simulink model "TST_HLSDem_SelectParameter"  (R2016b)
settings: Solver=FixedStepDiscrete  StartTime=0.0  StopTime=simTime  FixedStep=sampleTime  RelTol=1e-3
values from neighbouring files (symbols this model uses):
  testCase = 1    [initTST_HLSDem_SelectParameter_001.m]    (also in initTST_HLSDem_SelectParameter_002.m = 2; initTST_HLSDem_SelectParameter_003.m = 3; initTST_HLSDem_SelectParameter_004.m = 4; initTST_HLSDem_SelectParameter_005.m = 5)
libraries: simulink x146, UnitTest_Lib x140
(part 3 of 4)

== system TST_HLSDem_SelectParameter/simulationInput/testSignals_R002 ==
  BC : BusCreator  Inputs=37
  spec_CEngDsT_t : FromWorkspace  VariableName=testSig_CEngDsT_t  Interpolate=off  OutputAfterFinalValue=Holding final value
  spec_EngDa_tEng : FromWorkspace  VariableName=testSig_EngDa_tEng  Interpolate=off  OutputAfterFinalValue=Holding final value
  spec_Epm_nEng : FromWorkspace  VariableName=testSig_Epm_nEng  Interpolate=off  OutputAfterFinalValue=Holding final value
  spec_GlbDa_rTrqTot : FromWorkspace  VariableName=testSig_GlbDa_rTrqTot  Interpolate=off  OutputAfterFinalValue=Holding final value
  spec_HLSDem_IWinNegHiCurr_mp : FromWorkspace  VariableName=testSig_HLSDem_IWinNegHiCurr_mp  Interpolate=off  OutputAfterFinalValue=Holding final value
  spec_HLSDem_IWinNegLoCurr_mp : FromWorkspace  VariableName=testSig_HLSDem_IWinNegLoCurr_mp  Interpolate=off  OutputAfterFinalValue=Holding final value
  spec_HLSDem_IWinPosHiCurr_mp : FromWorkspace  VariableName=testSig_HLSDem_IWinPosHiCurr_mp  Interpolate=off  OutputAfterFinalValue=Holding final value
  spec_HLSDem_IWinPosLoCurr_mp : FromWorkspace  VariableName=testSig_HLSDem_IWinPosLoCurr_mp  Interpolate=off  OutputAfterFinalValue=Holding final value
  spec_HLSDem_InrtVehCurr : FromWorkspace  VariableName=testSig_HLSDem_InrtVehCurr  Interpolate=off  OutputAfterFinalValue=Holding final value
  spec_HLSDem_KiHiCurr_mp : FromWorkspace  VariableName=testSig_HLSDem_KiHiCurr_mp  Interpolate=off  OutputAfterFinalValue=Holding final value
  spec_HLSDem_KiLoCurr_mp : FromWorkspace  VariableName=testSig_HLSDem_KiLoCurr_mp  Interpolate=off  OutputAfterFinalValue=Holding final value
  spec_HLSDem_KiNegHiCurr_mp : FromWorkspace  VariableName=testSig_HLSDem_KiNegHiCurr_mp  Interpolate=off  OutputAfterFinalValue=Holding final value
  spec_HLSDem_KiNegLoCurr_mp : FromWorkspace  VariableName=testSig_HLSDem_KiNegLoCurr_mp  Interpolate=off  OutputAfterFinalValue=Holding final value
  spec_HLSDem_KiPosHiCurr_mp : FromWorkspace  VariableName=testSig_HLSDem_KiPosHiCurr_mp  Interpolate=off  OutputAfterFinalValue=Holding final value
  spec_HLSDem_KiPosLoCurr_mp : FromWorkspace  VariableName=testSig_HLSDem_KiPosLoCurr_mp  Interpolate=off  OutputAfterFinalValue=Holding final value
  spec_HLSDem_KpHiCurr_mp : FromWorkspace  VariableName=testSig_HLSDem_KpHiCurr_mp  Interpolate=off  OutputAfterFinalValue=Holding final value
  spec_HLSDem_KpLoCurr_mp : FromWorkspace  VariableName=testSig_HLSDem_KpLoCurr_mp  Interpolate=off  OutputAfterFinalValue=Holding final value
  spec_HLSDem_KpNegHiCurr_mp : FromWorkspace  VariableName=testSig_HLSDem_KpNegHiCurr_mp  Interpolate=off  OutputAfterFinalValue=Holding final value
  spec_HLSDem_KpNegLoCurr_mp : FromWorkspace  VariableName=testSig_HLSDem_KpNegLoCurr_mp  Interpolate=off  OutputAfterFinalValue=Holding final value
  spec_HLSDem_KpPosHiCurr_mp : FromWorkspace  VariableName=testSig_HLSDem_KpPosHiCurr_mp  Interpolate=off  OutputAfterFinalValue=Holding final value
  spec_HLSDem_KpPosLoCurr_mp : FromWorkspace  VariableName=testSig_HLSDem_KpPosLoCurr_mp  Interpolate=off  OutputAfterFinalValue=Holding final value
  spec_HLSDem_PWinNegHiCurr_mp : FromWorkspace  VariableName=testSig_HLSDem_PWinNegHiCurr_mp  Interpolate=off  OutputAfterFinalValue=Holding final value
  spec_HLSDem_PWinNegLoCurr_mp : FromWorkspace  VariableName=testSig_HLSDem_PWinNegLoCurr_mp  Interpolate=off  OutputAfterFinalValue=Holding final value
  spec_HLSDem_PWinPosHiCurr_mp : FromWorkspace  VariableName=testSig_HLSDem_PWinPosHiCurr_mp  Interpolate=off  OutputAfterFinalValue=Holding final value
  spec_HLSDem_PWinPosLoCurr_mp : FromWorkspace  VariableName=testSig_HLSDem_PWinPosLoCurr_mp  Interpolate=off  OutputAfterFinalValue=Holding final value
  spec_HLSDem_dnAccLim : FromWorkspace  VariableName=testSig_HLSDem_dnAccLim  Interpolate=off  OutputAfterFinalValue=Holding final value
  spec_HLSDem_dnDeclLim : FromWorkspace  VariableName=testSig_HLSDem_dnDeclLim  Interpolate=off  OutputAfterFinalValue=Holding final value
  spec_HLSDem_facFdbkHi : FromWorkspace  VariableName=testSig_HLSDem_facFdbkHi  Interpolate=off  OutputAfterFinalValue=Holding final value
  spec_HLSDem_facFdbkLo : FromWorkspace  VariableName=testSig_HLSDem_facFdbkLo  Interpolate=off  OutputAfterFinalValue=Holding final value
  spec_HLSDem_facFdbkTrqLosHi : FromWorkspace  VariableName=testSig_HLSDem_facFdbkTrqLosHi  Interpolate=off  OutputAfterFinalValue=Holding final value
  spec_HLSDem_facFdbkTrqLosLo : FromWorkspace  VariableName=testSig_HLSDem_facFdbkTrqLosLo  Interpolate=off  OutputAfterFinalValue=Holding final value
  spec_HLSDem_tiFltTrqLosEstCurr : FromWorkspace  VariableName=testSig_HLSDem_tiFltTrqLosEstCurr  Interpolate=off  OutputAfterFinalValue=Holding final value
  spec_Oil_tSwmp : FromWorkspace  VariableName=testSig_Oil_tSwmp  Interpolate=off  OutputAfterFinalValue=Holding final value
  spec_PT_rGrip : FromWorkspace  VariableName=testSig_PT_rGrip  Interpolate=off  OutputAfterFinalValue=Holding final value
  spec_PthLead_trqInrCurr : FromWorkspace  VariableName=testSig_PthLead_trqInrCurr  Interpolate=off  OutputAfterFinalValue=Holding final value
  spec_PthLead_trqInrLead : FromWorkspace  VariableName=testSig_PthLead_trqInrLead  Interpolate=off  OutputAfterFinalValue=Holding final value
  spec_PthSet_trqInrSet : FromWorkspace  VariableName=testSig_PthSet_trqInrSet  Interpolate=off  OutputAfterFinalValue=Holding final value
  testSignals : Outport
  wires:
  BC/1 -> testSignals/1
  spec_Epm_nEng/1 -> BC/1  "testSig_Epm_nEng"
  spec_PT_rGrip/1 -> BC/2  "testSig_PT_rGrip"
  spec_GlbDa_rTrqTot/1 -> BC/3  "testSig_GlbDa_rTrqTot"
  spec_PthSet_trqInrSet/1 -> BC/4  "testSig_PthSet_trqInrSet"
  spec_PthLead_trqInrCurr/1 -> BC/5  "testSig_PthLead_trqInrCurr"
  spec_PthLead_trqInrLead/1 -> BC/6  "testSig_PthLead_trqInrLead"
  spec_CEngDsT_t/1 -> BC/7  "testSig_CEngDsT_t"
  spec_Oil_tSwmp/1 -> BC/8  "testSig_Oil_tSwmp"
  spec_EngDa_tEng/1 -> BC/9  "testSig_EngDa_tEng"
  spec_HLSDem_facFdbkHi/1 -> BC/10  "testSig_HLSDem_facFdbkHi"
  spec_HLSDem_facFdbkLo/1 -> BC/11  "testSig_HLSDem_facFdbkLo"
  spec_HLSDem_facFdbkTrqLosLo/1 -> BC/12  "testSig_HLSDem_facFdbkTrqLosLo"
  spec_HLSDem_facFdbkTrqLosHi/1 -> BC/13  "testSig_HLSDem_facFdbkTrqLosHi"
  spec_HLSDem_tiFltTrqLosEstCurr/1 -> BC/14  "testSig_HLSDem_tiFltTrqLosEstCurr"
  spec_HLSDem_InrtVehCurr/1 -> BC/15  "testSig_HLSDem_InrtVehCurr"
  spec_HLSDem_dnAccLim/1 -> BC/16  "testSig_HLSDem_dnAccLim"
  spec_HLSDem_dnDeclLim/1 -> BC/17  "testSig_HLSDem_dnDeclLim"
  spec_HLSDem_KpLoCurr_mp/1 -> BC/18  "testSig_HLSDem_KpLoCurr_mp"
  spec_HLSDem_KpPosLoCurr_mp/1 -> BC/19  "testSig_HLSDem_KpPosLoCurr_mp"
  spec_HLSDem_KpNegLoCurr_mp/1 -> BC/20  "testSig_HLSDem_KpNegLoCurr_mp"
  spec_HLSDem_PWinPosLoCurr_mp/1 -> BC/21  "testSig_HLSDem_PWinPosLoCurr_mp"
  spec_HLSDem_PWinNegLoCurr_mp/1 -> BC/22  "testSig_HLSDem_PWinNegLoCurr_mp"
  spec_HLSDem_KiLoCurr_mp/1 -> BC/23  "testSig_HLSDem_KiLoCurr_mp"
  spec_HLSDem_KiPosLoCurr_mp/1 -> BC/24  "testSig_HLSDem_KiPosLoCurr_mp"
  spec_HLSDem_KiNegLoCurr_mp/1 -> BC/25  "testSig_HLSDem_KiNegLoCurr_mp"
  spec_HLSDem_IWinPosLoCurr_mp/1 -> BC/26  "testSig_HLSDem_IWinPosLoCurr_mp"
  spec_HLSDem_IWinNegLoCurr_mp/1 -> BC/27  "testSig_HLSDem_IWinNegLoCurr_mp"
  spec_HLSDem_KpHiCurr_mp/1 -> BC/28  "testSig_HLSDem_KpHiCurr_mp"
  spec_HLSDem_KpPosHiCurr_mp/1 -> BC/29  "testSig_HLSDem_KpPosHiCurr_mp"
  spec_HLSDem_KpNegHiCurr_mp/1 -> BC/30  "testSig_HLSDem_KpNegHiCurr_mp"
  spec_HLSDem_PWinPosHiCurr_mp/1 -> BC/31  "testSig_HLSDem_PWinPosHiCurr_mp"
  spec_HLSDem_PWinNegHiCurr_mp/1 -> BC/32  "testSig_HLSDem_PWinNegHiCurr_mp"
  spec_HLSDem_KiHiCurr_mp/1 -> BC/33  "testSig_HLSDem_KiHiCurr_mp"
  spec_HLSDem_KiPosHiCurr_mp/1 -> BC/34  "testSig_HLSDem_KiPosHiCurr_mp"
  spec_HLSDem_KiNegHiCurr_mp/1 -> BC/35  "testSig_HLSDem_KiNegHiCurr_mp"
  spec_HLSDem_IWinPosHiCurr_mp/1 -> BC/36  "testSig_HLSDem_IWinPosHiCurr_mp"
  spec_HLSDem_IWinNegHiCurr_mp/1 -> BC/37  "testSig_HLSDem_IWinNegHiCurr_mp"

== system TST_HLSDem_SelectParameter/simulationInput/testSignals_R003 ==
  BC : BusCreator  Inputs=37
  spec_CEngDsT_t : FromWorkspace  VariableName=testSig_CEngDsT_t  Interpolate=off  OutputAfterFinalValue=Holding final value
  spec_EngDa_tEng : FromWorkspace  VariableName=testSig_EngDa_tEng  Interpolate=off  OutputAfterFinalValue=Holding final value
  spec_Epm_nEng : FromWorkspace  VariableName=testSig_Epm_nEng  Interpolate=off  OutputAfterFinalValue=Holding final value
  spec_GlbDa_rTrqTot : FromWorkspace  VariableName=testSig_GlbDa_rTrqTot  Interpolate=off  OutputAfterFinalValue=Holding final value
  spec_HLSDem_IWinNegHiCurr_mp : FromWorkspace  VariableName=testSig_HLSDem_IWinNegHiCurr_mp  Interpolate=off  OutputAfterFinalValue=Holding final value
  spec_HLSDem_IWinNegLoCurr_mp : FromWorkspace  VariableName=testSig_HLSDem_IWinNegLoCurr_mp  Interpolate=off  OutputAfterFinalValue=Holding final value
  spec_HLSDem_IWinPosHiCurr_mp : FromWorkspace  VariableName=testSig_HLSDem_IWinPosHiCurr_mp  Interpolate=off  OutputAfterFinalValue=Holding final value
  spec_HLSDem_IWinPosLoCurr_mp : FromWorkspace  VariableName=testSig_HLSDem_IWinPosLoCurr_mp  Interpolate=off  OutputAfterFinalValue=Holding final value
  spec_HLSDem_InrtVehCurr : FromWorkspace  VariableName=testSig_HLSDem_InrtVehCurr  Interpolate=off  OutputAfterFinalValue=Holding final value
  spec_HLSDem_KiHiCurr_mp : FromWorkspace  VariableName=testSig_HLSDem_KiHiCurr_mp  Interpolate=off  OutputAfterFinalValue=Holding final value
  spec_HLSDem_KiLoCurr_mp : FromWorkspace  VariableName=testSig_HLSDem_KiLoCurr_mp  Interpolate=off  OutputAfterFinalValue=Holding final value
  spec_HLSDem_KiNegHiCurr_mp : FromWorkspace  VariableName=testSig_HLSDem_KiNegHiCurr_mp  Interpolate=off  OutputAfterFinalValue=Holding final value
  spec_HLSDem_KiNegLoCurr_mp : FromWorkspace  VariableName=testSig_HLSDem_KiNegLoCurr_mp  Interpolate=off  OutputAfterFinalValue=Holding final value
  spec_HLSDem_KiPosHiCurr_mp : FromWorkspace  VariableName=testSig_HLSDem_KiPosHiCurr_mp  Interpolate=off  OutputAfterFinalValue=Holding final value
  spec_HLSDem_KiPosLoCurr_mp : FromWorkspace  VariableName=testSig_HLSDem_KiPosLoCurr_mp  Interpolate=off  OutputAfterFinalValue=Holding final value
  spec_HLSDem_KpHiCurr_mp : FromWorkspace  VariableName=testSig_HLSDem_KpHiCurr_mp  Interpolate=off  OutputAfterFinalValue=Holding final value
  spec_HLSDem_KpLoCurr_mp : FromWorkspace  VariableName=testSig_HLSDem_KpLoCurr_mp  Interpolate=off  OutputAfterFinalValue=Holding final value
  spec_HLSDem_KpNegHiCurr_mp : FromWorkspace  VariableName=testSig_HLSDem_KpNegHiCurr_mp  Interpolate=off  OutputAfterFinalValue=Holding final value
  spec_HLSDem_KpNegLoCurr_mp : FromWorkspace  VariableName=testSig_HLSDem_KpNegLoCurr_mp  Interpolate=off  OutputAfterFinalValue=Holding final value
  spec_HLSDem_KpPosHiCurr_mp : FromWorkspace  VariableName=testSig_HLSDem_KpPosHiCurr_mp  Interpolate=off  OutputAfterFinalValue=Holding final value
  spec_HLSDem_KpPosLoCurr_mp : FromWorkspace  VariableName=testSig_HLSDem_KpPosLoCurr_mp  Interpolate=off  OutputAfterFinalValue=Holding final value
  spec_HLSDem_PWinNegHiCurr_mp : FromWorkspace  VariableName=testSig_HLSDem_PWinNegHiCurr_mp  Interpolate=off  OutputAfterFinalValue=Holding final value
  spec_HLSDem_PWinNegLoCurr_mp : FromWorkspace  VariableName=testSig_HLSDem_PWinNegLoCurr_mp  Interpolate=off  OutputAfterFinalValue=Holding final value
  spec_HLSDem_PWinPosHiCurr_mp : FromWorkspace  VariableName=testSig_HLSDem_PWinPosHiCurr_mp  Interpolate=off  OutputAfterFinalValue=Holding final value
  spec_HLSDem_PWinPosLoCurr_mp : FromWorkspace  VariableName=testSig_HLSDem_PWinPosLoCurr_mp  Interpolate=off  OutputAfterFinalValue=Holding final value
  spec_HLSDem_dnAccLim : FromWorkspace  VariableName=testSig_HLSDem_dnAccLim  Interpolate=off  OutputAfterFinalValue=Holding final value
  spec_HLSDem_dnDeclLim : FromWorkspace  VariableName=testSig_HLSDem_dnDeclLim  Interpolate=off  OutputAfterFinalValue=Holding final value
  spec_HLSDem_facFdbkHi : FromWorkspace  VariableName=testSig_HLSDem_facFdbkHi  Interpolate=off  OutputAfterFinalValue=Holding final value
  spec_HLSDem_facFdbkLo : FromWorkspace  VariableName=testSig_HLSDem_facFdbkLo  Interpolate=off  OutputAfterFinalValue=Holding final value
  spec_HLSDem_facFdbkTrqLosHi : FromWorkspace  VariableName=testSig_HLSDem_facFdbkTrqLosHi  Interpolate=off  OutputAfterFinalValue=Holding final value
  spec_HLSDem_facFdbkTrqLosLo : FromWorkspace  VariableName=testSig_HLSDem_facFdbkTrqLosLo  Interpolate=off  OutputAfterFinalValue=Holding final value
  spec_HLSDem_tiFltTrqLosEstCurr : FromWorkspace  VariableName=testSig_HLSDem_tiFltTrqLosEstCurr  Interpolate=off  OutputAfterFinalValue=Holding final value
  spec_Oil_tSwmp : FromWorkspace  VariableName=testSig_Oil_tSwmp  Interpolate=off  OutputAfterFinalValue=Holding final value
  spec_PT_rGrip : FromWorkspace  VariableName=testSig_PT_rGrip  Interpolate=off  OutputAfterFinalValue=Holding final value
  spec_PthLead_trqInrCurr : FromWorkspace  VariableName=testSig_PthLead_trqInrCurr  Interpolate=off  OutputAfterFinalValue=Holding final value
  spec_PthLead_trqInrLead : FromWorkspace  VariableName=testSig_PthLead_trqInrLead  Interpolate=off  OutputAfterFinalValue=Holding final value
  spec_PthSet_trqInrSet : FromWorkspace  VariableName=testSig_PthSet_trqInrSet  Interpolate=off  OutputAfterFinalValue=Holding final value
  testSignals : Outport
  wires:
  BC/1 -> testSignals/1
  spec_Epm_nEng/1 -> BC/1  "testSig_Epm_nEng"
  spec_PT_rGrip/1 -> BC/2  "testSig_PT_rGrip"
  spec_GlbDa_rTrqTot/1 -> BC/3  "testSig_GlbDa_rTrqTot"
  spec_PthSet_trqInrSet/1 -> BC/4  "testSig_PthSet_trqInrSet"
  spec_PthLead_trqInrCurr/1 -> BC/5  "testSig_PthLead_trqInrCurr"
  spec_PthLead_trqInrLead/1 -> BC/6  "testSig_PthLead_trqInrLead"
  spec_CEngDsT_t/1 -> BC/7  "testSig_CEngDsT_t"
  spec_Oil_tSwmp/1 -> BC/8  "testSig_Oil_tSwmp"
  spec_EngDa_tEng/1 -> BC/9  "testSig_EngDa_tEng"
  spec_HLSDem_facFdbkHi/1 -> BC/10  "testSig_HLSDem_facFdbkHi"
  spec_HLSDem_facFdbkLo/1 -> BC/11  "testSig_HLSDem_facFdbkLo"
  spec_HLSDem_facFdbkTrqLosLo/1 -> BC/12  "testSig_HLSDem_facFdbkTrqLosLo"
  spec_HLSDem_facFdbkTrqLosHi/1 -> BC/13  "testSig_HLSDem_facFdbkTrqLosHi"
  spec_HLSDem_tiFltTrqLosEstCurr/1 -> BC/14  "testSig_HLSDem_tiFltTrqLosEstCurr"
  spec_HLSDem_InrtVehCurr/1 -> BC/15  "testSig_HLSDem_InrtVehCurr"
  spec_HLSDem_dnAccLim/1 -> BC/16  "testSig_HLSDem_dnAccLim"
  spec_HLSDem_dnDeclLim/1 -> BC/17  "testSig_HLSDem_dnDeclLim"
  spec_HLSDem_KpLoCurr_mp/1 -> BC/18  "testSig_HLSDem_KpLoCurr_mp"
  spec_HLSDem_KpPosLoCurr_mp/1 -> BC/19  "testSig_HLSDem_KpPosLoCurr_mp"
  spec_HLSDem_KpNegLoCurr_mp/1 -> BC/20  "testSig_HLSDem_KpNegLoCurr_mp"
  spec_HLSDem_PWinPosLoCurr_mp/1 -> BC/21  "testSig_HLSDem_PWinPosLoCurr_mp"
  spec_HLSDem_PWinNegLoCurr_mp/1 -> BC/22  "testSig_HLSDem_PWinNegLoCurr_mp"
  spec_HLSDem_KiLoCurr_mp/1 -> BC/23  "testSig_HLSDem_KiLoCurr_mp"
  spec_HLSDem_KiPosLoCurr_mp/1 -> BC/24  "testSig_HLSDem_KiPosLoCurr_mp"
  spec_HLSDem_KiNegLoCurr_mp/1 -> BC/25  "testSig_HLSDem_KiNegLoCurr_mp"
  spec_HLSDem_IWinPosLoCurr_mp/1 -> BC/26  "testSig_HLSDem_IWinPosLoCurr_mp"
  spec_HLSDem_IWinNegLoCurr_mp/1 -> BC/27  "testSig_HLSDem_IWinNegLoCurr_mp"
  spec_HLSDem_KpHiCurr_mp/1 -> BC/28  "testSig_HLSDem_KpHiCurr_mp"
  spec_HLSDem_KpPosHiCurr_mp/1 -> BC/29  "testSig_HLSDem_KpPosHiCurr_mp"
  spec_HLSDem_KpNegHiCurr_mp/1 -> BC/30  "testSig_HLSDem_KpNegHiCurr_mp"
  spec_HLSDem_PWinPosHiCurr_mp/1 -> BC/31  "testSig_HLSDem_PWinPosHiCurr_mp"
  spec_HLSDem_PWinNegHiCurr_mp/1 -> BC/32  "testSig_HLSDem_PWinNegHiCurr_mp"
  spec_HLSDem_KiHiCurr_mp/1 -> BC/33  "testSig_HLSDem_KiHiCurr_mp"
  spec_HLSDem_KiPosHiCurr_mp/1 -> BC/34  "testSig_HLSDem_KiPosHiCurr_mp"
  spec_HLSDem_KiNegHiCurr_mp/1 -> BC/35  "testSig_HLSDem_KiNegHiCurr_mp"
  spec_HLSDem_IWinPosHiCurr_mp/1 -> BC/36  "testSig_HLSDem_IWinPosHiCurr_mp"
  spec_HLSDem_IWinNegHiCurr_mp/1 -> BC/37  "testSig_HLSDem_IWinNegHiCurr_mp"

== system TST_HLSDem_SelectParameter/simulationInput/testSignals_R004 ==
  BC : BusCreator  Inputs=37
  spec_CEngDsT_t : FromWorkspace  VariableName=testSig_CEngDsT_t  Interpolate=off  OutputAfterFinalValue=Holding final value
  spec_EngDa_tEng : FromWorkspace  VariableName=testSig_EngDa_tEng  Interpolate=off  OutputAfterFinalValue=Holding final value
  spec_Epm_nEng : FromWorkspace  VariableName=testSig_Epm_nEng  Interpolate=off  OutputAfterFinalValue=Holding final value
  spec_GlbDa_rTrqTot : FromWorkspace  VariableName=testSig_GlbDa_rTrqTot  Interpolate=off  OutputAfterFinalValue=Holding final value
  spec_HLSDem_IWinNegHiCurr_mp : FromWorkspace  VariableName=testSig_HLSDem_IWinNegHiCurr_mp  Interpolate=off  OutputAfterFinalValue=Holding final value
  spec_HLSDem_IWinNegLoCurr_mp : FromWorkspace  VariableName=testSig_HLSDem_IWinNegLoCurr_mp  Interpolate=off  OutputAfterFinalValue=Holding final value
  spec_HLSDem_IWinPosHiCurr_mp : FromWorkspace  VariableName=testSig_HLSDem_IWinPosHiCurr_mp  Interpolate=off  OutputAfterFinalValue=Holding final value
  spec_HLSDem_IWinPosLoCurr_mp : FromWorkspace  VariableName=testSig_HLSDem_IWinPosLoCurr_mp  Interpolate=off  OutputAfterFinalValue=Holding final value
  spec_HLSDem_InrtVehCurr : FromWorkspace  VariableName=testSig_HLSDem_InrtVehCurr  Interpolate=off  OutputAfterFinalValue=Holding final value
  spec_HLSDem_KiHiCurr_mp : FromWorkspace  VariableName=testSig_HLSDem_KiHiCurr_mp  Interpolate=off  OutputAfterFinalValue=Holding final value
  spec_HLSDem_KiLoCurr_mp : FromWorkspace  VariableName=testSig_HLSDem_KiLoCurr_mp  Interpolate=off  OutputAfterFinalValue=Holding final value
  spec_HLSDem_KiNegHiCurr_mp : FromWorkspace  VariableName=testSig_HLSDem_KiNegHiCurr_mp  Interpolate=off  OutputAfterFinalValue=Holding final value
  spec_HLSDem_KiNegLoCurr_mp : FromWorkspace  VariableName=testSig_HLSDem_KiNegLoCurr_mp  Interpolate=off  OutputAfterFinalValue=Holding final value
  spec_HLSDem_KiPosHiCurr_mp : FromWorkspace  VariableName=testSig_HLSDem_KiPosHiCurr_mp  Interpolate=off  OutputAfterFinalValue=Holding final value
  spec_HLSDem_KiPosLoCurr_mp : FromWorkspace  VariableName=testSig_HLSDem_KiPosLoCurr_mp  Interpolate=off  OutputAfterFinalValue=Holding final value
  spec_HLSDem_KpHiCurr_mp : FromWorkspace  VariableName=testSig_HLSDem_KpHiCurr_mp  Interpolate=off  OutputAfterFinalValue=Holding final value
  spec_HLSDem_KpLoCurr_mp : FromWorkspace  VariableName=testSig_HLSDem_KpLoCurr_mp  Interpolate=off  OutputAfterFinalValue=Holding final value
  spec_HLSDem_KpNegHiCurr_mp : FromWorkspace  VariableName=testSig_HLSDem_KpNegHiCurr_mp  Interpolate=off  OutputAfterFinalValue=Holding final value
  spec_HLSDem_KpNegLoCurr_mp : FromWorkspace  VariableName=testSig_HLSDem_KpNegLoCurr_mp  Interpolate=off  OutputAfterFinalValue=Holding final value
  spec_HLSDem_KpPosHiCurr_mp : FromWorkspace  VariableName=testSig_HLSDem_KpPosHiCurr_mp  Interpolate=off  OutputAfterFinalValue=Holding final value
  spec_HLSDem_KpPosLoCurr_mp : FromWorkspace  VariableName=testSig_HLSDem_KpPosLoCurr_mp  Interpolate=off  OutputAfterFinalValue=Holding final value
  spec_HLSDem_PWinNegHiCurr_mp : FromWorkspace  VariableName=testSig_HLSDem_PWinNegHiCurr_mp  Interpolate=off  OutputAfterFinalValue=Holding final value
  spec_HLSDem_PWinNegLoCurr_mp : FromWorkspace  VariableName=testSig_HLSDem_PWinNegLoCurr_mp  Interpolate=off  OutputAfterFinalValue=Holding final value
  spec_HLSDem_PWinPosHiCurr_mp : FromWorkspace  VariableName=testSig_HLSDem_PWinPosHiCurr_mp  Interpolate=off  OutputAfterFinalValue=Holding final value
  spec_HLSDem_PWinPosLoCurr_mp : FromWorkspace  VariableName=testSig_HLSDem_PWinPosLoCurr_mp  Interpolate=off  OutputAfterFinalValue=Holding final value
  spec_HLSDem_dnAccLim : FromWorkspace  VariableName=testSig_HLSDem_dnAccLim  Interpolate=off  OutputAfterFinalValue=Holding final value
  spec_HLSDem_dnDeclLim : FromWorkspace  VariableName=testSig_HLSDem_dnDeclLim  Interpolate=off  OutputAfterFinalValue=Holding final value
  spec_HLSDem_facFdbkHi : FromWorkspace  VariableName=testSig_HLSDem_facFdbkHi  Interpolate=off  OutputAfterFinalValue=Holding final value
  spec_HLSDem_facFdbkLo : FromWorkspace  VariableName=testSig_HLSDem_facFdbkLo  Interpolate=off  OutputAfterFinalValue=Holding final value
  spec_HLSDem_facFdbkTrqLosHi : FromWorkspace  VariableName=testSig_HLSDem_facFdbkTrqLosHi  Interpolate=off  OutputAfterFinalValue=Holding final value
  spec_HLSDem_facFdbkTrqLosLo : FromWorkspace  VariableName=testSig_HLSDem_facFdbkTrqLosLo  Interpolate=off  OutputAfterFinalValue=Holding final value
  spec_HLSDem_tiFltTrqLosEstCurr : FromWorkspace  VariableName=testSig_HLSDem_tiFltTrqLosEstCurr  Interpolate=off  OutputAfterFinalValue=Holding final value
  spec_Oil_tSwmp : FromWorkspace  VariableName=testSig_Oil_tSwmp  Interpolate=off  OutputAfterFinalValue=Holding final value
  spec_PT_rGrip : FromWorkspace  VariableName=testSig_PT_rGrip  Interpolate=off  OutputAfterFinalValue=Holding final value
  spec_PthLead_trqInrCurr : FromWorkspace  VariableName=testSig_PthLead_trqInrCurr  Interpolate=off  OutputAfterFinalValue=Holding final value
  spec_PthLead_trqInrLead : FromWorkspace  VariableName=testSig_PthLead_trqInrLead  Interpolate=off  OutputAfterFinalValue=Holding final value
  spec_PthSet_trqInrSet : FromWorkspace  VariableName=testSig_PthSet_trqInrSet  Interpolate=off  OutputAfterFinalValue=Holding final value
  testSignals : Outport
  wires:
  BC/1 -> testSignals/1
  spec_Epm_nEng/1 -> BC/1  "testSig_Epm_nEng"
  spec_PT_rGrip/1 -> BC/2  "testSig_PT_rGrip"
  spec_GlbDa_rTrqTot/1 -> BC/3  "testSig_GlbDa_rTrqTot"
  spec_PthSet_trqInrSet/1 -> BC/4  "testSig_PthSet_trqInrSet"
  spec_PthLead_trqInrCurr/1 -> BC/5  "testSig_PthLead_trqInrCurr"
  spec_PthLead_trqInrLead/1 -> BC/6  "testSig_PthLead_trqInrLead"
  spec_CEngDsT_t/1 -> BC/7  "testSig_CEngDsT_t"
  spec_Oil_tSwmp/1 -> BC/8  "testSig_Oil_tSwmp"
  spec_EngDa_tEng/1 -> BC/9  "testSig_EngDa_tEng"
  spec_HLSDem_facFdbkHi/1 -> BC/10  "testSig_HLSDem_facFdbkHi"
  spec_HLSDem_facFdbkLo/1 -> BC/11  "testSig_HLSDem_facFdbkLo"
  spec_HLSDem_facFdbkTrqLosLo/1 -> BC/12  "testSig_HLSDem_facFdbkTrqLosLo"
  spec_HLSDem_facFdbkTrqLosHi/1 -> BC/13  "testSig_HLSDem_facFdbkTrqLosHi"
  spec_HLSDem_tiFltTrqLosEstCurr/1 -> BC/14  "testSig_HLSDem_tiFltTrqLosEstCurr"
  spec_HLSDem_InrtVehCurr/1 -> BC/15  "testSig_HLSDem_InrtVehCurr"
  spec_HLSDem_dnAccLim/1 -> BC/16  "testSig_HLSDem_dnAccLim"
  spec_HLSDem_dnDeclLim/1 -> BC/17  "testSig_HLSDem_dnDeclLim"
  spec_HLSDem_KpLoCurr_mp/1 -> BC/18  "testSig_HLSDem_KpLoCurr_mp"
  spec_HLSDem_KpPosLoCurr_mp/1 -> BC/19  "testSig_HLSDem_KpPosLoCurr_mp"
  spec_HLSDem_KpNegLoCurr_mp/1 -> BC/20  "testSig_HLSDem_KpNegLoCurr_mp"
  spec_HLSDem_PWinPosLoCurr_mp/1 -> BC/21  "testSig_HLSDem_PWinPosLoCurr_mp"
  spec_HLSDem_PWinNegLoCurr_mp/1 -> BC/22  "testSig_HLSDem_PWinNegLoCurr_mp"
  spec_HLSDem_KiLoCurr_mp/1 -> BC/23  "testSig_HLSDem_KiLoCurr_mp"
  spec_HLSDem_KiPosLoCurr_mp/1 -> BC/24  "testSig_HLSDem_KiPosLoCurr_mp"
  spec_HLSDem_KiNegLoCurr_mp/1 -> BC/25  "testSig_HLSDem_KiNegLoCurr_mp"
  spec_HLSDem_IWinPosLoCurr_mp/1 -> BC/26  "testSig_HLSDem_IWinPosLoCurr_mp"
  spec_HLSDem_IWinNegLoCurr_mp/1 -> BC/27  "testSig_HLSDem_IWinNegLoCurr_mp"
  spec_HLSDem_KpHiCurr_mp/1 -> BC/28  "testSig_HLSDem_KpHiCurr_mp"
  spec_HLSDem_KpPosHiCurr_mp/1 -> BC/29  "testSig_HLSDem_KpPosHiCurr_mp"
  spec_HLSDem_KpNegHiCurr_mp/1 -> BC/30  "testSig_HLSDem_KpNegHiCurr_mp"
  spec_HLSDem_PWinPosHiCurr_mp/1 -> BC/31  "testSig_HLSDem_PWinPosHiCurr_mp"
  spec_HLSDem_PWinNegHiCurr_mp/1 -> BC/32  "testSig_HLSDem_PWinNegHiCurr_mp"
  spec_HLSDem_KiHiCurr_mp/1 -> BC/33  "testSig_HLSDem_KiHiCurr_mp"
  spec_HLSDem_KiPosHiCurr_mp/1 -> BC/34  "testSig_HLSDem_KiPosHiCurr_mp"
  spec_HLSDem_KiNegHiCurr_mp/1 -> BC/35  "testSig_HLSDem_KiNegHiCurr_mp"
  spec_HLSDem_IWinPosHiCurr_mp/1 -> BC/36  "testSig_HLSDem_IWinPosHiCurr_mp"
  spec_HLSDem_IWinNegHiCurr_mp/1 -> BC/37  "testSig_HLSDem_IWinNegHiCurr_mp"

== system TST_HLSDem_SelectParameter/simulationInput/testSignals_R005 ==
  BC : BusCreator  Inputs=37
  spec_CEngDsT_t : FromWorkspace  VariableName=testSig_CEngDsT_t  Interpolate=off  OutputAfterFinalValue=Holding final value
  spec_EngDa_tEng : FromWorkspace  VariableName=testSig_EngDa_tEng  Interpolate=off  OutputAfterFinalValue=Holding final value
  spec_Epm_nEng : FromWorkspace  VariableName=testSig_Epm_nEng  Interpolate=off  OutputAfterFinalValue=Holding final value
  spec_GlbDa_rTrqTot : FromWorkspace  VariableName=testSig_GlbDa_rTrqTot  Interpolate=off  OutputAfterFinalValue=Holding final value
  spec_HLSDem_IWinNegHiCurr_mp : FromWorkspace  VariableName=testSig_HLSDem_IWinNegHiCurr_mp  Interpolate=off  OutputAfterFinalValue=Holding final value
  spec_HLSDem_IWinNegLoCurr_mp : FromWorkspace  VariableName=testSig_HLSDem_IWinNegLoCurr_mp  Interpolate=off  OutputAfterFinalValue=Holding final value
  spec_HLSDem_IWinPosHiCurr_mp : FromWorkspace  VariableName=testSig_HLSDem_IWinPosHiCurr_mp  Interpolate=off  OutputAfterFinalValue=Holding final value
  spec_HLSDem_IWinPosLoCurr_mp : FromWorkspace  VariableName=testSig_HLSDem_IWinPosLoCurr_mp  Interpolate=off  OutputAfterFinalValue=Holding final value
  spec_HLSDem_InrtVehCurr : FromWorkspace  VariableName=testSig_HLSDem_InrtVehCurr  Interpolate=off  OutputAfterFinalValue=Holding final value
  spec_HLSDem_KiHiCurr_mp : FromWorkspace  VariableName=testSig_HLSDem_KiHiCurr_mp  Interpolate=off  OutputAfterFinalValue=Holding final value
  spec_HLSDem_KiLoCurr_mp : FromWorkspace  VariableName=testSig_HLSDem_KiLoCurr_mp  Interpolate=off  OutputAfterFinalValue=Holding final value
  spec_HLSDem_KiNegHiCurr_mp : FromWorkspace  VariableName=testSig_HLSDem_KiNegHiCurr_mp  Interpolate=off  OutputAfterFinalValue=Holding final value
  spec_HLSDem_KiNegLoCurr_mp : FromWorkspace  VariableName=testSig_HLSDem_KiNegLoCurr_mp  Interpolate=off  OutputAfterFinalValue=Holding final value
  spec_HLSDem_KiPosHiCurr_mp : FromWorkspace  VariableName=testSig_HLSDem_KiPosHiCurr_mp  Interpolate=off  OutputAfterFinalValue=Holding final value
  spec_HLSDem_KiPosLoCurr_mp : FromWorkspace  VariableName=testSig_HLSDem_KiPosLoCurr_mp  Interpolate=off  OutputAfterFinalValue=Holding final value
  spec_HLSDem_KpHiCurr_mp : FromWorkspace  VariableName=testSig_HLSDem_KpHiCurr_mp  Interpolate=off  OutputAfterFinalValue=Holding final value
  spec_HLSDem_KpLoCurr_mp : FromWorkspace  VariableName=testSig_HLSDem_KpLoCurr_mp  Interpolate=off  OutputAfterFinalValue=Holding final value
  spec_HLSDem_KpNegHiCurr_mp : FromWorkspace  VariableName=testSig_HLSDem_KpNegHiCurr_mp  Interpolate=off  OutputAfterFinalValue=Holding final value
  spec_HLSDem_KpNegLoCurr_mp : FromWorkspace  VariableName=testSig_HLSDem_KpNegLoCurr_mp  Interpolate=off  OutputAfterFinalValue=Holding final value
  spec_HLSDem_KpPosHiCurr_mp : FromWorkspace  VariableName=testSig_HLSDem_KpPosHiCurr_mp  Interpolate=off  OutputAfterFinalValue=Holding final value
  spec_HLSDem_KpPosLoCurr_mp : FromWorkspace  VariableName=testSig_HLSDem_KpPosLoCurr_mp  Interpolate=off  OutputAfterFinalValue=Holding final value
  spec_HLSDem_PWinNegHiCurr_mp : FromWorkspace  VariableName=testSig_HLSDem_PWinNegHiCurr_mp  Interpolate=off  OutputAfterFinalValue=Holding final value
  spec_HLSDem_PWinNegLoCurr_mp : FromWorkspace  VariableName=testSig_HLSDem_PWinNegLoCurr_mp  Interpolate=off  OutputAfterFinalValue=Holding final value
  spec_HLSDem_PWinPosHiCurr_mp : FromWorkspace  VariableName=testSig_HLSDem_PWinPosHiCurr_mp  Interpolate=off  OutputAfterFinalValue=Holding final value
  spec_HLSDem_PWinPosLoCurr_mp : FromWorkspace  VariableName=testSig_HLSDem_PWinPosLoCurr_mp  Interpolate=off  OutputAfterFinalValue=Holding final value
  spec_HLSDem_dnAccLim : FromWorkspace  VariableName=testSig_HLSDem_dnAccLim  Interpolate=off  OutputAfterFinalValue=Holding final value
  spec_HLSDem_dnDeclLim : FromWorkspace  VariableName=testSig_HLSDem_dnDeclLim  Interpolate=off  OutputAfterFinalValue=Holding final value
  spec_HLSDem_facFdbkHi : FromWorkspace  VariableName=testSig_HLSDem_facFdbkHi  Interpolate=off  OutputAfterFinalValue=Holding final value
  spec_HLSDem_facFdbkLo : FromWorkspace  VariableName=testSig_HLSDem_facFdbkLo  Interpolate=off  OutputAfterFinalValue=Holding final value
  spec_HLSDem_facFdbkTrqLosHi : FromWorkspace  VariableName=testSig_HLSDem_facFdbkTrqLosHi  Interpolate=off  OutputAfterFinalValue=Holding final value
  spec_HLSDem_facFdbkTrqLosLo : FromWorkspace  VariableName=testSig_HLSDem_facFdbkTrqLosLo  Interpolate=off  OutputAfterFinalValue=Holding final value
  spec_HLSDem_tiFltTrqLosEstCurr : FromWorkspace  VariableName=testSig_HLSDem_tiFltTrqLosEstCurr  Interpolate=off  OutputAfterFinalValue=Holding final value
  spec_Oil_tSwmp : FromWorkspace  VariableName=testSig_Oil_tSwmp  Interpolate=off  OutputAfterFinalValue=Holding final value
  spec_PT_rGrip : FromWorkspace  VariableName=testSig_PT_rGrip  Interpolate=off  OutputAfterFinalValue=Holding final value
  spec_PthLead_trqInrCurr : FromWorkspace  VariableName=testSig_PthLead_trqInrCurr  Interpolate=off  OutputAfterFinalValue=Holding final value
  spec_PthLead_trqInrLead : FromWorkspace  VariableName=testSig_PthLead_trqInrLead  Interpolate=off  OutputAfterFinalValue=Holding final value
  spec_PthSet_trqInrSet : FromWorkspace  VariableName=testSig_PthSet_trqInrSet  Interpolate=off  OutputAfterFinalValue=Holding final value
  testSignals : Outport
  wires:
  BC/1 -> testSignals/1
  spec_Epm_nEng/1 -> BC/1  "testSig_Epm_nEng"
  spec_PT_rGrip/1 -> BC/2  "testSig_PT_rGrip"
  spec_GlbDa_rTrqTot/1 -> BC/3  "testSig_GlbDa_rTrqTot"
  spec_PthSet_trqInrSet/1 -> BC/4  "testSig_PthSet_trqInrSet"
  spec_PthLead_trqInrCurr/1 -> BC/5  "testSig_PthLead_trqInrCurr"
  spec_PthLead_trqInrLead/1 -> BC/6  "testSig_PthLead_trqInrLead"
  spec_CEngDsT_t/1 -> BC/7  "testSig_CEngDsT_t"
  spec_Oil_tSwmp/1 -> BC/8  "testSig_Oil_tSwmp"
  spec_EngDa_tEng/1 -> BC/9  "testSig_EngDa_tEng"
  spec_HLSDem_facFdbkHi/1 -> BC/10  "testSig_HLSDem_facFdbkHi"
  spec_HLSDem_facFdbkLo/1 -> BC/11  "testSig_HLSDem_facFdbkLo"
  spec_HLSDem_facFdbkTrqLosLo/1 -> BC/12  "testSig_HLSDem_facFdbkTrqLosLo"
  spec_HLSDem_facFdbkTrqLosHi/1 -> BC/13  "testSig_HLSDem_facFdbkTrqLosHi"
  spec_HLSDem_tiFltTrqLosEstCurr/1 -> BC/14  "testSig_HLSDem_tiFltTrqLosEstCurr"
  spec_HLSDem_InrtVehCurr/1 -> BC/15  "testSig_HLSDem_InrtVehCurr"
  spec_HLSDem_dnAccLim/1 -> BC/16  "testSig_HLSDem_dnAccLim"
  spec_HLSDem_dnDeclLim/1 -> BC/17  "testSig_HLSDem_dnDeclLim"
  spec_HLSDem_KpLoCurr_mp/1 -> BC/18  "testSig_HLSDem_KpLoCurr_mp"
  spec_HLSDem_KpPosLoCurr_mp/1 -> BC/19  "testSig_HLSDem_KpPosLoCurr_mp"
  spec_HLSDem_KpNegLoCurr_mp/1 -> BC/20  "testSig_HLSDem_KpNegLoCurr_mp"
  spec_HLSDem_PWinPosLoCurr_mp/1 -> BC/21  "testSig_HLSDem_PWinPosLoCurr_mp"
  spec_HLSDem_PWinNegLoCurr_mp/1 -> BC/22  "testSig_HLSDem_PWinNegLoCurr_mp"
  spec_HLSDem_KiLoCurr_mp/1 -> BC/23  "testSig_HLSDem_KiLoCurr_mp"
  spec_HLSDem_KiPosLoCurr_mp/1 -> BC/24  "testSig_HLSDem_KiPosLoCurr_mp"
  spec_HLSDem_KiNegLoCurr_mp/1 -> BC/25  "testSig_HLSDem_KiNegLoCurr_mp"
  spec_HLSDem_IWinPosLoCurr_mp/1 -> BC/26  "testSig_HLSDem_IWinPosLoCurr_mp"
  spec_HLSDem_IWinNegLoCurr_mp/1 -> BC/27  "testSig_HLSDem_IWinNegLoCurr_mp"
  spec_HLSDem_KpHiCurr_mp/1 -> BC/28  "testSig_HLSDem_KpHiCurr_mp"
  spec_HLSDem_KpPosHiCurr_mp/1 -> BC/29  "testSig_HLSDem_KpPosHiCurr_mp"
  spec_HLSDem_KpNegHiCurr_mp/1 -> BC/30  "testSig_HLSDem_KpNegHiCurr_mp"
  spec_HLSDem_PWinPosHiCurr_mp/1 -> BC/31  "testSig_HLSDem_PWinPosHiCurr_mp"
  spec_HLSDem_PWinNegHiCurr_mp/1 -> BC/32  "testSig_HLSDem_PWinNegHiCurr_mp"
  spec_HLSDem_KiHiCurr_mp/1 -> BC/33  "testSig_HLSDem_KiHiCurr_mp"
  spec_HLSDem_KiPosHiCurr_mp/1 -> BC/34  "testSig_HLSDem_KiPosHiCurr_mp"
  spec_HLSDem_KiNegHiCurr_mp/1 -> BC/35  "testSig_HLSDem_KiNegHiCurr_mp"
  spec_HLSDem_IWinPosHiCurr_mp/1 -> BC/36  "testSig_HLSDem_IWinPosHiCurr_mp"
  spec_HLSDem_IWinNegHiCurr_mp/1 -> BC/37  "testSig_HLSDem_IWinNegHiCurr_mp"

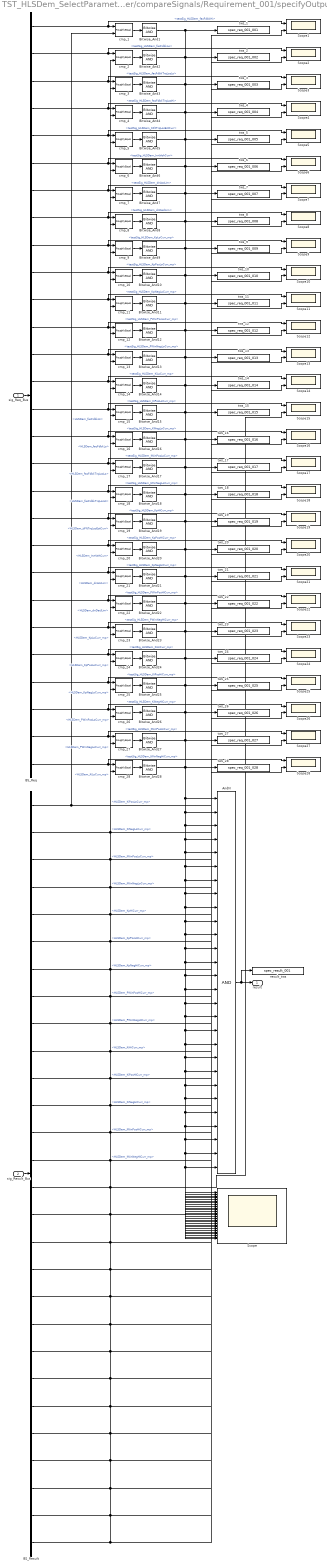
== system TST_HLSDem_SelectParameter/compareSignals/Requirement_001/specifyOutputs ==
  sig_Req_Bus : Inport
  sig_Result_Bus : Inport  Port=2
  AndN : Logic  Inputs=28
  BS_Req : BusSelector  OutputSignals=testSig_HLSDem_facFdbkHi,testSig_HLSDem_facFdbkLo,testSig_HLSDem_facFdbkTrqLosLo,testSig_HLSDem_facFdbkTrqLosHi,testSig_HLSDem_tiFltTrqLosEstCurr,testSig_HLSDem_InrtVehCurr,testSig_HLSDem_dnAccLim,testSig_HLSDem_dnDeclLim,testSig_HLSDem_KpLoCurr_mp,testSig_HLSDem_KpPosLoCurr_mp,testSig_HLSDem_KpNegLoCurr_mp,testSig_HLSDem_PWinPosLoCurr_mp,testSig_HLSDem_PWinNegLoCurr_mp,testSig_HLSDem_KiLoCurr_mp,testSig_HLSDem_KiPosLoCurr_mp,testSig_HLSDem_KiNegLoCurr_mp,testSig_HLSDem_IWinPosLoCurr_mp,testSig_HLSDem_IWinNegLoCurr_mp,testSig_HLSDem_KpHiCurr_mp,testSig_HLSDem_KpPosHiCurr_mp,testSig_HLSDem_KpNegHiCurr_mp,testSig_HLSDem_PWinPosHiCurr_mp,testSig_HLSDem_PWinNegHiCurr_mp,testSig_HLSDem_KiHiCurr_mp,testSig_HLSDem_KiPosHiCurr_mp,testSig_HLSDem_KiNegHiCurr_mp,testSig_HLSDem_IWinPosHiCurr_mp,testSig_HLSDem_IWinNegHiCurr_mp
  BS_Result : BusSelector  OutputSignals=HLSDem_facFdbkHi,HLSDem_facFdbkLo,HLSDem_facFdbkTrqLosLo,HLSDem_facFdbkTrqLosHi,HLSDem_tiFltTrqLosEstCurr,HLSDem_InrtVehCurr,HLSDem_dnAccLim,HLSDem_dnDeclLim,HLSDem_KpLoCurr_mp,HLSDem_KpPosLoCurr_mp,HLSDem_KpNegLoCurr_mp,HLSDem_PWinPosLoCurr_mp,HLSDem_PWinNegLoCurr_mp,HLSDem_KiLoCurr_mp,HLSDem_KiPosLoCurr_mp,HLSDem_KiNegLoCurr_mp,HLSDem_IWinPosLoCurr_mp,HLSDem_IWinNegLoCurr_mp,HLSDem_KpHiCurr_mp,HLSDem_KpPosHiCurr_mp,HLSDem_KpNegHiCurr_mp,HLSDem_PWinPosHiCurr_mp,HLSDem_PWinNegHiCurr_mp,HLSDem_KiHiCurr_mp,HLSDem_KiPosHiCurr_mp,HLSDem_KiNegHiCurr_mp,HLSDem_IWinPosHiCurr_mp,HLSDem_IWinNegHiCurr_mp
  Bitwise_And{1..28} (28 alike) : simulink/Logic and Bit Operations/Bitwise Operator  logicop=AND  UseBitMask=off  BitMask=bin2dec('11011001')  BitMaskRealWorld=Stored Integer
  Scope : Scope  NumInputPorts=28
  Scope{1..28} (28 alike) : Scope  NumInputPorts=2
  cmp_{1..6,9..28} (26 alike) : UnitTest_Lib/RoughlyEqual  slope=0.1
  cmp_7 : UnitTest_Lib/RoughlyEqual  slope=1
  cmp_8 : UnitTest_Lib/RoughlyEqual  slope=1
  result_tws : ToWorkspace  VariableName=spec_result_001
  tws_1 : ToWorkspace  VariableName=spec_req_001_001
  tws_10 : ToWorkspace  VariableName=spec_req_001_010
  tws_11 : ToWorkspace  VariableName=spec_req_001_011
  tws_12 : ToWorkspace  VariableName=spec_req_001_012
  tws_13 : ToWorkspace  VariableName=spec_req_001_013
  tws_14 : ToWorkspace  VariableName=spec_req_001_014
  tws_15 : ToWorkspace  VariableName=spec_req_001_015
  tws_16 : ToWorkspace  VariableName=spec_req_001_016
  tws_17 : ToWorkspace  VariableName=spec_req_001_017
  tws_18 : ToWorkspace  VariableName=spec_req_001_018
  tws_19 : ToWorkspace  VariableName=spec_req_001_019
  tws_2 : ToWorkspace  VariableName=spec_req_001_002
  tws_20 : ToWorkspace  VariableName=spec_req_001_020
  tws_21 : ToWorkspace  VariableName=spec_req_001_021
  tws_22 : ToWorkspace  VariableName=spec_req_001_022
  tws_23 : ToWorkspace  VariableName=spec_req_001_023
  tws_24 : ToWorkspace  VariableName=spec_req_001_024
  tws_25 : ToWorkspace  VariableName=spec_req_001_025
  tws_26 : ToWorkspace  VariableName=spec_req_001_026
  tws_27 : ToWorkspace  VariableName=spec_req_001_027
  tws_28 : ToWorkspace  VariableName=spec_req_001_028
  tws_3 : ToWorkspace  VariableName=spec_req_001_003
  tws_4 : ToWorkspace  VariableName=spec_req_001_004
  tws_5 : ToWorkspace  VariableName=spec_req_001_005
  tws_6 : ToWorkspace  VariableName=spec_req_001_006
  tws_7 : ToWorkspace  VariableName=spec_req_001_007
  tws_8 : ToWorkspace  VariableName=spec_req_001_008
  tws_9 : ToWorkspace  VariableName=spec_req_001_009
  result : Outport
  wires:
  sig_Req_Bus/1 -> BS_Req/1
  sig_Result_Bus/1 -> BS_Result/1
  AndN/1 -> result/1, result_tws/1
  BS_Req/1 -> cmp_1/1, Scope1/1  "<testSig_HLSDem_facFdbkHi>"
  BS_Result/1 -> cmp_1/2, Scope1/2  "<HLSDem_facFdbkHi>"
  cmp_1/1 -> Bitwise_And1/1
  Bitwise_And1/1 -> AndN/1, Scope/1, tws_1/1
  BS_Req/2 -> cmp_2/1, Scope2/1  "<testSig_HLSDem_facFdbkLo>"
  BS_Result/2 -> cmp_2/2, Scope2/2  "<HLSDem_facFdbkLo>"
  cmp_2/1 -> Bitwise_And2/1
  Bitwise_And2/1 -> AndN/2, Scope/2, tws_2/1
  BS_Req/3 -> cmp_3/1, Scope3/1  "<testSig_HLSDem_facFdbkTrqLosLo>"
  BS_Result/3 -> cmp_3/2, Scope3/2  "<HLSDem_facFdbkTrqLosLo>"
  cmp_3/1 -> Bitwise_And3/1
  Bitwise_And3/1 -> AndN/3, Scope/3, tws_3/1
  BS_Req/4 -> cmp_4/1, Scope4/1  "<testSig_HLSDem_facFdbkTrqLosHi>"
  BS_Result/4 -> cmp_4/2, Scope4/2  "<HLSDem_facFdbkTrqLosHi>"
  cmp_4/1 -> Bitwise_And4/1
  Bitwise_And4/1 -> AndN/4, Scope/4, tws_4/1
  BS_Req/5 -> cmp_5/1, Scope5/1  "<testSig_HLSDem_tiFltTrqLosEstCurr>"
  BS_Result/5 -> cmp_5/2, Scope5/2  "<HLSDem_tiFltTrqLosEstCurr>"
  cmp_5/1 -> Bitwise_And5/1
  Bitwise_And5/1 -> AndN/5, Scope/5, tws_5/1
  BS_Req/6 -> cmp_6/1, Scope6/1  "<testSig_HLSDem_InrtVehCurr>"
  BS_Result/6 -> cmp_6/2, Scope6/2  "<HLSDem_InrtVehCurr>"
  cmp_6/1 -> Bitwise_And6/1
  Bitwise_And6/1 -> AndN/6, Scope/6, tws_6/1
  BS_Req/7 -> cmp_7/1, Scope7/1  "<testSig_HLSDem_dnAccLim>"
  BS_Result/7 -> cmp_7/2, Scope7/2  "<HLSDem_dnAccLim>"
  cmp_7/1 -> Bitwise_And7/1
  Bitwise_And7/1 -> AndN/7, Scope/7, tws_7/1
  BS_Req/8 -> cmp_8/1, Scope8/1  "<testSig_HLSDem_dnDeclLim>"
  BS_Result/8 -> cmp_8/2, Scope8/2  "<HLSDem_dnDeclLim>"
  cmp_8/1 -> Bitwise_And8/1
  Bitwise_And8/1 -> AndN/8, Scope/8, tws_8/1
  BS_Req/9 -> cmp_9/1, Scope9/1  "<testSig_HLSDem_KpLoCurr_mp>"
  BS_Result/9 -> cmp_9/2, Scope9/2  "<HLSDem_KpLoCurr_mp>"
  cmp_9/1 -> Bitwise_And9/1
  Bitwise_And9/1 -> AndN/9, Scope/9, tws_9/1
  BS_Req/10 -> cmp_10/1, Scope10/1  "<testSig_HLSDem_KpPosLoCurr_mp>"
  BS_Result/10 -> cmp_10/2, Scope10/2  "<HLSDem_KpPosLoCurr_mp>"
  cmp_10/1 -> Bitwise_And10/1
  Bitwise_And10/1 -> AndN/10, Scope/10, tws_10/1
  BS_Req/11 -> cmp_11/1, Scope11/1  "<testSig_HLSDem_KpNegLoCurr_mp>"
  BS_Result/11 -> cmp_11/2, Scope11/2  "<HLSDem_KpNegLoCurr_mp>"
  cmp_11/1 -> Bitwise_And11/1
  Bitwise_And11/1 -> AndN/11, Scope/11, tws_11/1
  BS_Req/12 -> cmp_12/1, Scope12/1  "<testSig_HLSDem_PWinPosLoCurr_mp>"
  BS_Result/12 -> cmp_12/2, Scope12/2  "<HLSDem_PWinPosLoCurr_mp>"
  cmp_12/1 -> Bitwise_And12/1
  Bitwise_And12/1 -> AndN/12, Scope/12, tws_12/1
  BS_Req/13 -> cmp_13/1, Scope13/1  "<testSig_HLSDem_PWinNegLoCurr_mp>"
  BS_Result/13 -> cmp_13/2, Scope13/2  "<HLSDem_PWinNegLoCurr_mp>"
  cmp_13/1 -> Bitwise_And13/1
  Bitwise_And13/1 -> AndN/13, Scope/13, tws_13/1
  BS_Req/14 -> cmp_14/1, Scope14/1  "<testSig_HLSDem_KiLoCurr_mp>"
  BS_Result/14 -> cmp_14/2, Scope14/2  "<HLSDem_KiLoCurr_mp>"
  cmp_14/1 -> Bitwise_And14/1
  Bitwise_And14/1 -> AndN/14, Scope/14, tws_14/1
  BS_Req/15 -> cmp_15/1, Scope15/1  "<testSig_HLSDem_KiPosLoCurr_mp>"
  BS_Result/15 -> cmp_15/2, Scope15/2  "<HLSDem_KiPosLoCurr_mp>"
  cmp_15/1 -> Bitwise_And15/1
  Bitwise_And15/1 -> AndN/15, Scope/15, tws_15/1
  BS_Req/16 -> cmp_16/1, Scope16/1  "<testSig_HLSDem_KiNegLoCurr_mp>"
  BS_Result/16 -> cmp_16/2, Scope16/2  "<HLSDem_KiNegLoCurr_mp>"
  cmp_16/1 -> Bitwise_And16/1
  Bitwise_And16/1 -> AndN/16, Scope/16, tws_16/1
  BS_Req/17 -> cmp_17/1, Scope17/1  "<testSig_HLSDem_IWinPosLoCurr_mp>"
  BS_Result/17 -> cmp_17/2, Scope17/2  "<HLSDem_IWinPosLoCurr_mp>"
  cmp_17/1 -> Bitwise_And17/1
  Bitwise_And17/1 -> AndN/17, Scope/17, tws_17/1
  BS_Req/18 -> cmp_18/1, Scope18/1  "<testSig_HLSDem_IWinNegLoCurr_mp>"
  BS_Result/18 -> cmp_18/2, Scope18/2  "<HLSDem_IWinNegLoCurr_mp>"
  cmp_18/1 -> Bitwise_And18/1
  Bitwise_And18/1 -> AndN/18, Scope/18, tws_18/1
  BS_Req/19 -> cmp_19/1, Scope19/1  "<testSig_HLSDem_KpHiCurr_mp>"
  BS_Result/19 -> cmp_19/2, Scope19/2  "<HLSDem_KpHiCurr_mp>"
  cmp_19/1 -> Bitwise_And19/1
  Bitwise_And19/1 -> AndN/19, Scope/19, tws_19/1
  BS_Req/20 -> cmp_20/1, Scope20/1  "<testSig_HLSDem_KpPosHiCurr_mp>"
  BS_Result/20 -> cmp_20/2, Scope20/2  "<HLSDem_KpPosHiCurr_mp>"
  cmp_20/1 -> Bitwise_And20/1
  Bitwise_And20/1 -> AndN/20, Scope/20, tws_20/1
  BS_Req/21 -> cmp_21/1, Scope21/1  "<testSig_HLSDem_KpNegHiCurr_mp>"
  BS_Result/21 -> cmp_21/2, Scope21/2  "<HLSDem_KpNegHiCurr_mp>"
  cmp_21/1 -> Bitwise_And21/1
  Bitwise_And21/1 -> AndN/21, Scope/21, tws_21/1
  BS_Req/22 -> cmp_22/1, Scope22/1  "<testSig_HLSDem_PWinPosHiCurr_mp>"
  BS_Result/22 -> cmp_22/2, Scope22/2  "<HLSDem_PWinPosHiCurr_mp>"
  cmp_22/1 -> Bitwise_And22/1
  Bitwise_And22/1 -> AndN/22, Scope/22, tws_22/1
  BS_Req/23 -> cmp_23/1, Scope23/1  "<testSig_HLSDem_PWinNegHiCurr_mp>"
  BS_Result/23 -> cmp_23/2, Scope23/2  "<HLSDem_PWinNegHiCurr_mp>"
  cmp_23/1 -> Bitwise_And23/1
  Bitwise_And23/1 -> AndN/23, Scope/23, tws_23/1
  BS_Req/24 -> cmp_24/1, Scope24/1  "<testSig_HLSDem_KiHiCurr_mp>"
  BS_Result/24 -> cmp_24/2, Scope24/2  "<HLSDem_KiHiCurr_mp>"
  cmp_24/1 -> Bitwise_And24/1
  Bitwise_And24/1 -> AndN/24, Scope/24, tws_24/1
  BS_Req/25 -> cmp_25/1, Scope25/1  "<testSig_HLSDem_KiPosHiCurr_mp>"
  BS_Result/25 -> cmp_25/2, Scope25/2  "<HLSDem_KiPosHiCurr_mp>"
  cmp_25/1 -> Bitwise_And25/1
  Bitwise_And25/1 -> AndN/25, Scope/25, tws_25/1
  BS_Req/26 -> cmp_26/1, Scope26/1  "<testSig_HLSDem_KiNegHiCurr_mp>"
  BS_Result/26 -> cmp_26/2, Scope26/2  "<HLSDem_KiNegHiCurr_mp>"
  cmp_26/1 -> Bitwise_And26/1
  Bitwise_And26/1 -> AndN/26, Scope/26, tws_26/1
  BS_Req/27 -> cmp_27/1, Scope27/1  "<testSig_HLSDem_IWinPosHiCurr_mp>"
  BS_Result/27 -> cmp_27/2, Scope27/2  "<HLSDem_IWinPosHiCurr_mp>"
  cmp_27/1 -> Bitwise_And27/1
  Bitwise_And27/1 -> AndN/27, Scope/27, tws_27/1
  BS_Req/28 -> cmp_28/1, Scope28/1  "<testSig_HLSDem_IWinNegHiCurr_mp>"
  BS_Result/28 -> cmp_28/2, Scope28/2  "<HLSDem_IWinNegHiCurr_mp>"
  cmp_28/1 -> Bitwise_And28/1
  Bitwise_And28/1 -> AndN/28, Scope/28, tws_28/1
